simulink model "EjemSFun_2019"  (R2021a)
settings: Solver=VariableStepAuto  StartTime=0.0  StopTime=10  FixedStep=100e-3  MaxStep=1e-3  RelTol=1e-3
settings Model: SimulationMode=accelerator  Creator=david  LastModifiedBy=kenny
settings SolverCC: AlgebraicLoopSolver=TrustRegion
settings DebuggingCC: SFMachineParentedDataDiag=warning

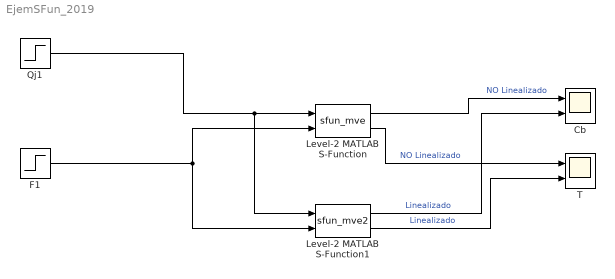
== system EjemSFun_2019 ==
  Cb : Scope  NumInputPorts=2
  F1 : Step  Time=3  Before=141.9  After=145  SampleTime=0
  Level-2 MATLAB S-Function : M-S-Function  FunctionName=sfun_mve  Parameters=[2.1304 1.0903 387.34 386.06]
  Level-2 MATLAB S-Function1 : M-S-Function  FunctionName=sfun_mve2  Parameters=[2.1304 1.0903 387.34 386.06]
  Qj1 : Step  Time=5  Before=-1113.5  After=-1500  SampleTime=0
  T : Scope  NumInputPorts=2
  wires:
  Level-2 MATLAB S-Function/1 -> Cb/1  "NO Linealizado"
  Level-2 MATLAB S-Function/2 -> T/1  "NO Linealizado"
  Level-2 MATLAB S-Function1/1 -> Cb/2  "Linealizado"
  Level-2 MATLAB S-Function1/2 -> T/2  "Linealizado"
  Qj1/1 -> Level-2 MATLAB S-Function1/1, Level-2 MATLAB S-Function/1
  F1/1 -> Level-2 MATLAB S-Function/2, Level-2 MATLAB S-Function1/2
